simulink model "ML_UAV_3D_2"  (R2018a)
settings: Solver=ode4  StartTime=0.0  StopTime=130  FixedStep=Ts  MaxStep=2*T  MinStep=T  RelTol=1e-4
values from neighbouring files (symbols this model uses):
  Ac = 0.0331    [init_ML_UAV_3D_2.m]
  Am1_LPF = sysd.denominator{1}    [init_ML_UAV_3D_2.m]
  Am2_LPF = sysd.denominator{1}    [init_ML_UAV_3D_2.m]
  Am_coup_LPF = sysd.denominator{1}    [init_ML_UAV_3D_2.m]
  Amp_sf = 3    [init_ML_UAV_3D_2.m]
  Amp_sf_rp = 0.05*uav.m*g    [init_ML_UAV_3D_2.m]
  Bm1_LPF = sysd.numerator{1}    [init_ML_UAV_3D_2.m]
  Bm2_LPF = sysd.numerator{1}    [init_ML_UAV_3D_2.m]
  Bm_coup_LPF = sysd.numerator{1}    [init_ML_UAV_3D_2.m]
  C_S = [5;5;9]*10^-3    [init_ML_UAV_3D_2.m]
  Cd_u = 0.2    [init_ML_UAV_3D_2.m]
  dc_M_p = 6.7    [init_ML_UAV_3D_2.m]
  eps_V = 0.5    [init_ML_UAV_3D_2.m]
  g = 9.81    [init_ML_UAV_3D_2.m]
  gamma_d_p = (2*0.3/0.03*2*0.2*12/4)/10    (= 2.4)    [init_ML_UAV_3D_2.m]
  k3 = 24    [init_ML_UAV_3D_2.m]
  k4 = 0.8    [init_ML_UAV_3D_2.m]
  min_sf = 5    [init_ML_UAV_3D_2.m]
  min_sf_rp = 0.35*uav.m*g    [init_ML_UAV_3D_2.m]
  OMEGA_FILTER_OUTER = 40    [estimation.m]
  T_init = 10    [init_ML_UAV_3D_2.m]
  Tc = 1/500    (= 0.002)    [estimation.m]
  Tg = 1/ 20    (= 0.05)    [estimation.m]
  Tn = 1/500    (= 0.002)    [estimation.m]
  Ts = 1/500    (= 0.002)    [estimation.m]    (also in init_ML_UAV_3D_2.m)
  Tsc = 1/100    (= 0.01)    [estimation.m]
  Tz = 1/500    (= 0.002)    [estimation.m]
  X_GPS_offset = [0.01 0.005]    [estimation.m]
undefined symbols (not defined in the file or in its folder): Am_HPF, Am_LPF, Am_LPF2, an1, an1_v, an2, an3, Bm_HPF, Bm_LPF, Bm_LPF2, bn1, bn1_v, bn2, bn3, buoy, cable, controller, current, D_b, DiscIntNeverNeededParam, F, filters, J_u, K, kd_t, kp_t, L, Light, magnitude, MIL, Phi0, Psi0, R_b, T, Theta0, theta_q_ini, tolerences, torque_corr, uav, Vol_b, water, wave, X0_u
libraries: simulink x48, simulink_extras x10, UAV_Control x4, dspmtrx3 x2, aerolibwind2 x2
(part 5 of 6)

== system ML_UAV_3D_2/Quadrotor+buoy/6-DOF equations of motion Earth frame/M_1-5/buoy inertia ==
  Rb : Inport
  Rb_T : Inport  Port=2
  Demux : Demux  Outputs=3
  Demux1 : Demux  Outputs=2
  M_ii{,1..3} (4 alike) : Scope
  Product1 : Product  Inputs=3  Multiplication=Matrix(*)
  Selector : Selector  NumberOfDimensions=2  InputPortWidth=3  IndexOptions=Index vector (dialog),Index vector (dialog)  Indices=[1],[1 2 3]  OutputSizes=1,1
  Selector1 : Selector  NumberOfDimensions=2  InputPortWidth=3  IndexOptions=Index vector (dialog),Index vector (dialog)  Indices=[2],[2 3]  OutputSizes=1,1
  Selector2 : Selector  NumberOfDimensions=2  InputPortWidth=3  IndexOptions=Index vector (dialog),Index vector (dialog)  Indices=[3],[3]  OutputSizes=1,1
  Sum : Sum  Inputs=|++
  added mass : Constant  Value=diag([a_ii(1), a_ii(2), a_ii(3)])
  rigid body mass : Constant  Value=diag([m_b,m_b,m_b])
  M11_I : Outport
  M22_I : Outport  Port=2
  M12_I : Outport  Port=3
  M13_I : Outport  Port=4
  M33_I : Outport  Port=5
  M23_I : Outport  Port=6
  wires:
  rigid body mass/1 -> Sum/1
  added mass/1 -> Sum/2
  Rb/1 -> Product1/1  "Rb"
  Sum/1 -> Product1/2  "Mb'"
  Selector2/1 -> M_ii2/1, M33_I/1
  Selector/1 -> M_ii/1, Demux/1
  Product1/1 -> Selector2/1, Selector1/1, M_ii3/1, Selector/1
  Selector1/1 -> M_ii1/1, Demux1/1
  Demux/1 -> M11_I/1
  Demux/2 -> M12_I/1
  Demux/3 -> M13_I/1
  Demux1/1 -> M22_I/1
  Demux1/2 -> M23_I/1
  Rb_T/1 -> Product1/3

== system ML_UAV_3D_2/Quadrotor+buoy/6-DOF equations of motion Earth frame/M_12/added mass ==
  theta : Inport
  Add1 : Sum
  Add2 : Sum
  Add3 : Sum  Inputs=+-
  Constant13 : Constant  Value=2
  Gain : Gain  Gain=2
  M11 : Constant  Value=m_b+a_ii(1)
  "M11 " : Constant  Value=m_b+a_ii(1)
  M11 1 : Constant  Value=m_b+a_ii(1)
  "M22 " : Constant  Value=m_b+a_ii(2)
  M22 1 : Constant  Value=m_b+a_ii(2)
  M_22 : Constant  Value=m_b+a_ii(2)
  Product{,6..8} (4 alike) : Product  Inputs=3
  Product9 : Product  Inputs=**/
  Trigonometric Function1 : Trigonometry  Operator=sincos
  Trigonometric Function2 : Trigonometry  Operator=sincos
  Trigonometric Function3 : Trigonometry
  M11_I : Outport
  M22_I : Outport  Port=2
  M12_I : Outport  Port=3
  wires:
  Gain/1 -> Trigonometric Function3/1
  "M11 "/1 -> Product7/1
  Constant13/1 -> Product9/3
  Product7/1 -> Add2/1
  Add3/1 -> Product9/2
  M11 1/1 -> Add3/2
  M11/1 -> Product6/3
  M22 1/1 -> Add3/1
  "M22 "/1 -> Product8/3
  Product/1 -> Add1/1
  Product6/1 -> Add1/2
  Add2/1 -> M22_I/1
  Product8/1 -> Add2/2
  Trigonometric Function1/2 -> Product6/2, Product6/1
  Trigonometric Function2/1 -> Product7/3, Product7/2
  Trigonometric Function2/2 -> Product8/1, Product8/2
  M_22/1 -> Product/1
  Trigonometric Function3/1 -> Product9/1
  Trigonometric Function1/1 -> Product/2, Product/3
  theta/1 -> Gain/1, Trigonometric Function2/1, Trigonometric Function1/1
  Product9/1 -> M12_I/1
  Add1/1 -> M11_I/1

== system ML_UAV_3D_2/Quadrotor+buoy/6-DOF equations of motion Earth frame/Quadrotor Dynamics Outer-Loop/Gu ==
  coupled : Inport
  Constant4 : Constant  Value=m_u
  Gain1 : Gain  Gain=g
  Ground : Ground
  Product : Product
  Vector Concatenate : Concatenate  NumInputs=3
  G : Outport
  wires:
  Product/1 -> Gain1/1
  Constant4/1 -> Product/2  "u2"
  coupled/1 -> Product/1
  Vector Concatenate/1 -> G/1
  Gain1/1 -> Vector Concatenate/3  "u2"
  Ground/1 -> Vector Concatenate/2, Vector Concatenate/1

== system ML_UAV_3D_2/Quadrotor+buoy/6-DOF equations of motion Earth frame/Quadrotor Dynamics Outer-Loop/Integrator while decoupled ==
  acc : Inport
  X dot init : Inport  Port=2
  X init : Inport  Port=3
  X123 : Inport  Port=4
  reset : Inport  Port=5
  Enable : EnablePort
  Bias : Bias  Bias=L
  Bias3 : Bias  Bias=-L
  Saturation Dynamic : simulink/Discontinuities/Saturation Dynamic  OutMin=[]  OutMax=[]  OutDataTypeStr=Inherit: Same as second input  OutDataType=fixdt(1, 16)  OutScaling=2^-10  DoSatur=off
  Selector : Selector  InputPortWidth=5  IndexOptions=Index vector (dialog)  Indices=[1 2 3]  OutputSizes=1
  Selector1 : Selector  InputPortWidth=5  IndexOptions=Index vector (dialog)  Indices=[1 2 3]  OutputSizes=1
  Vector Concatenate2 : Concatenate
  Xu : DiscreteIntegrator  IntegratorMethod=Integration: Backward Euler  ExternalReset=level  InitialConditionSource=external  InitialCondition=theta_q_ini  SampleTime=-1  LimitOutput=on  StateName=theta  ICPrevOutput=DiscIntNeverNeededParam  ICPrevScaledInput=DiscIntNeverNeededParam
  dot(Xu) : DiscreteIntegrator  IntegratorMethod=Integration: Backward Euler  gainval=1  ExternalReset=level  InitialConditionSource=external  SampleTime=-1  ICPrevOutput=DiscIntNeverNeededParam  ICPrevScaledInput=DiscIntNeverNeededParam
  theta u{1..10} (10 alike) : Scope
  "dot(Xu) " : Outport
  "Xu " : Outport  Port=2
  wires:
  X dot init/1 -> theta u5/1, dot(Xu)/3
  Xu/1 -> theta u6/1, Vector Concatenate2/1, Saturation Dynamic/2
  X init/1 -> theta u7/1, Xu/3
  Saturation Dynamic/1 -> Vector Concatenate2/2, "Xu "/1
  X123/1 -> Selector/1, Selector1/1
  Selector/1 -> Bias/1
  Bias3/1 -> theta u10/1, Saturation Dynamic/3
  Vector Concatenate2/1 -> theta u3/1
  Bias/1 -> Saturation Dynamic/1, theta u9/1
  dot(Xu)/1 -> Xu/1, theta u1/1, "dot(Xu) "/1
  reset/1 -> theta u2/1, dot(Xu)/2, Xu/2
  acc/1 -> theta u4/1, dot(Xu)/1
  Selector1/1 -> theta u8/1, Bias3/1

== system ML_UAV_3D_2/Quadrotor+buoy/6-DOF equations of motion Earth frame/Quadrotor Dynamics Outer-Loop/Subsystem ==
  u1 : Inport
  R_u_3 : Inport  Port=2
  Product1 : Product  Inputs=**  SaturateOnIntegerOverflow=on  InputSameDT=on  OutDataTypeStr=Inherit: Same as first input
  tau_u : Outport
  wires:
  Product1/1 -> tau_u/1
  R_u_3/1 -> Product1/1
  u1/1 -> Product1/2

== system ML_UAV_3D_2/Quadrotor+buoy/6-DOF equations of motion Earth frame/Quadrotor Dynamics Outer-Loop/get initial UAV states for the decoupled dynamics ==
  X : Inport
  Xdot : Inport  Port=2
  Trigger : TriggerPort  TriggerType=falling  VariantControl=Variant
  Xu_init : Outport
  Vu_init : Outport  Port=2
  wires:
  X/1 -> Xu_init/1
  Xdot/1 -> Vu_init/1

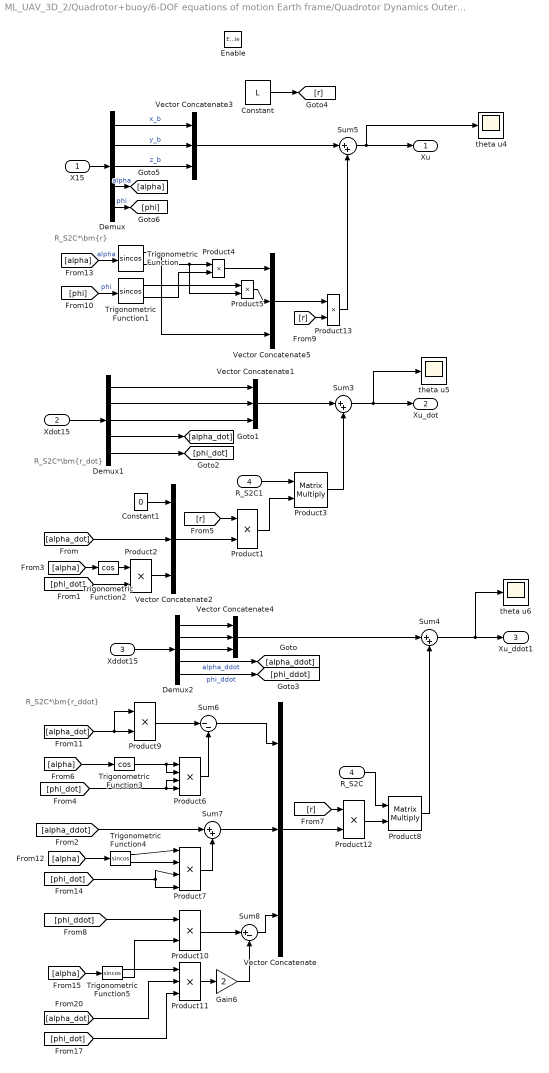
== system ML_UAV_3D_2/Quadrotor+buoy/6-DOF equations of motion Earth frame/Quadrotor Dynamics Outer-Loop/quadrotor position from relative buoy-UAV position ==
  note: R_S2C*\bm{r_ddot}
  note: R_S2C*\bm{r_dot}
  note: R_S2C*\bm{r}
  X15 : Inport
  Xdot15 : Inport  Port=2
  Xddot15 : Inport  Port=3
  R_S2C : Inport  Port=4
  Enable : EnablePort
  Constant : Constant  Value=L
  Constant1 : Constant  Value=0
  Demux : Demux  Outputs=5
  Demux1 : Demux  Outputs=5
  Demux2 : Demux  Outputs=5
  Gain6 : Gain  Gain=2
  Product{1..2,4..5,9..10,12..13} (8 alike) : Product
  Product11 : Product  Inputs=3
  Product3 : Product  Multiplication=Matrix(*)
  Product6 : Product  Inputs=4
  Product7 : Product  Inputs=4
  Product8 : Product  Multiplication=Matrix(*)
  R_S2C1 : InportShadow  Port=4
  Sum{3..5,7} (4 alike) : Sum  Inputs=|++
  Sum6 : Sum  Inputs=|--
  Sum8 : Sum  Inputs=|+-
  Trigonometric Function{,1,4..5} (4 alike) : Trigonometry  Operator=sincos
  Trigonometric Function2 : Trigonometry  Operator=cos
  Trigonometric Function3 : Trigonometry  Operator=cos
  Vector Concatenate{,1..5} (6 alike) : Concatenate  NumInputs=3
  theta u4 : Scope
  theta u5 : Scope
  theta u6 : Scope
  Xu : Outport
  Xu_dot : Outport  Port=2
  Xu_ddot1 : Outport  Port=3
  wires:
  [alpha] -> Trigonometric Function/1  "alpha"
  Sum5/1 -> Xu/1, theta u4/1
  Trigonometric Function/2 -> Product5/2, Product4/1
  Demux/2 -> Vector Concatenate3/2  "y_b"
  X15/1 -> Demux/1
  Demux/1 -> Vector Concatenate3/1  "x_b"
  R_S2C1/1 -> Product3/1
  Xdot15/1 -> Demux1/1
  Demux1/1 -> Vector Concatenate1/1
  Sum3/1 -> Xu_dot/1, theta u5/1
  Demux1/3 -> Vector Concatenate1/3
  Xddot15/1 -> Demux2/1
  Demux2/4 -> [alpha_ddot]  "alpha_ddot"
  [alpha_dot] -> Vector Concatenate2/2
  Product1/1 -> Product3/2
  Sum4/1 -> theta u6/1, Xu_ddot1/1
  Demux2/1 -> Vector Concatenate4/1
  Demux2/2 -> Vector Concatenate4/2
  [phi] -> Trigonometric Function1/1  "phi"
  Trigonometric Function1/2 -> Product4/2
  Trigonometric Function1/1 -> Product5/1
  Demux2/3 -> Vector Concatenate4/3
  [phi_dot] -> Product11/3
  Sum7/1 -> Vector Concatenate/2
  Product10/1 -> Sum8/1
  Vector Concatenate/1 -> Product12/2
  [alpha_dot] -> Product11/2
  [alpha] -> Trigonometric Function4/1
  Product7/1 -> Sum7/2
  Sum6/1 -> Vector Concatenate/1
  Sum8/1 -> Vector Concatenate/3
  Product6/1 -> Sum6/2
  Product11/1 -> Gain6/1
  Trigonometric Function5/1 -> Product11/1
  [alpha] -> Trigonometric Function5/1
  Product9/1 -> Sum6/1
  [alpha] -> Trigonometric Function3/1
  Demux2/5 -> [phi_ddot]  "phi_ddot"
  Demux1/5 -> [phi_dot]
  Demux1/4 -> [alpha_dot]
  Demux1/2 -> Vector Concatenate1/2
  Constant/1 -> [r]
  [alpha_ddot] -> Sum7/1
  [phi_ddot] -> Product10/1
  Trigonometric Function5/2 -> Product10/2
  Gain6/1 -> Sum8/2
  [r] -> Product12/1
  [alpha_dot] -> Product9/2, Product9/1
  Trigonometric Function3/1 -> Product6/2, Product6/1
  [phi_dot] -> Product6/3, Product6/4
  Trigonometric Function4/1 -> Product7/1
  Trigonometric Function4/2 -> Product7/2
  [phi_dot] -> Product7/4, Product7/3
  Product12/1 -> Product8/2
  R_S2C/1 -> Product8/1
  Vector Concatenate4/1 -> Sum4/1
  Product8/1 -> Sum4/2
  Constant1/1 -> Vector Concatenate2/1
  Product2/1 -> Vector Concatenate2/3
  [phi_dot] -> Product2/2
  [alpha] -> Trigonometric Function2/1
  Trigonometric Function2/1 -> Product2/1
  [r] -> Product1/1
  Vector Concatenate2/1 -> Product1/2
  Vector Concatenate1/1 -> Sum3/1
  Product3/1 -> Sum3/2
  Demux/3 -> Vector Concatenate3/3  "z_b"
  Vector Concatenate3/1 -> Sum5/1
  Product13/1 -> Sum5/2
  Product4/1 -> Vector Concatenate5/1
  Product5/1 -> Vector Concatenate5/2
  Trigonometric Function/1 -> Vector Concatenate5/3
  Vector Concatenate5/1 -> Product13/1
  [r] -> Product13/2
  Demux/4 -> [alpha]  "alpha"
  Demux/5 -> [phi]  "phi"

== system ML_UAV_3D_2/Quadrotor+buoy/6-DOF equations of motion Earth frame/Rigid Body Torque Equations /Rotation Angles to Angular transformation matrix body to earth Rotation Order: ZXY ==
  R1,R2,R3 : Inport  PortDimensions=3
  Fcn1 : Fcn  Expr=0
  Fcn11 : Fcn  Expr=u(5)
  Fcn13 : Fcn  Expr=u(2)
  Fcn21 : Fcn  Expr=u(2)*u(1)/u(4)
  Fcn22 : Fcn  Expr=1
  Fcn23 : Fcn  Expr=-u(5)*u(1)/u(4)
  Fcn3 : Fcn  Expr=u(5)/u(4)
  Fcn32 : Fcn  Expr=0
  Fcn33 : Fcn  Expr=-u(2)/u(4)
  Mux : Mux  Inputs=2
  Subsystem : Subsystem
  sincos : Trigonometry  Operator=sincos
  T : Outport  PortDimensions=[3,3]
  wires:
  R1,R2,R3/1 -> sincos/1
  Subsystem/1(Out1) -> T/1
  sincos/1 -> Mux/1
  sincos/2 -> Mux/2
  Mux/1 -> Fcn22/1, Fcn33/1, Fcn21/1, Fcn11/1, Fcn32/1, Fcn13/1, Fcn23/1, Fcn3/1, Fcn1/1
  Fcn11/1 -> Subsystem/1(In1)
  Fcn21/1 -> Subsystem/2(In2)
  Fcn33/1 -> Subsystem/3(In3)
  Fcn32/1 -> Subsystem/4(In4)
  Fcn13/1 -> Subsystem/7(In7)
  Fcn22/1 -> Subsystem/5(In5)
  Fcn1/1 -> Subsystem/6(In6)
  Fcn23/1 -> Subsystem/8(In8)
  Fcn3/1 -> Subsystem/9(In9)

== system ML_UAV_3D_2/Quadrotor+buoy/6-DOF equations of motion Earth frame/Tension from UAV, X and r directions/Tension from UAV, z direction ==
  alpha : Inport
  euler_u : Inport  Port=2
  u1 : Inport  Port=3
  Xu_ddot : Inport  Port=4
  Enable : EnablePort  StatesWhenEnabling=reset
  Add3 : Sum  Inputs=+--
  Constant : Constant  Value=m_u*g
  Demux : Demux  Outputs=2
  Gain14 : Gain
  Gain15 : Gain  Gain=m_u
  Product12 : Product  Inputs=3
  Product9 : Product  Inputs=*/
  Trigonometric Function6 : Trigonometry
  Trigonometric Function8 : Trigonometry  Operator=cos
  "phi, theta" : Selector  InputPortWidth=3  IndexOptions=Index vector (dialog)  Indices=[1 2]  OutputSizes=1
  z_ddot : Selector  InputPortWidth=3  IndexOptions=Index vector (dialog)  Indices=3  OutputSizes=1
  "T, from z simple" : Outport
  wires:
  Product9/1 -> "T, from z simple"/1
  Add3/1 -> Product9/1
  Gain14/1 -> Add3/1
  Demux/1 -> Product12/1
  u1/1 -> Product12/3
  alpha/1 -> Trigonometric Function6/1
  Product12/1 -> Gain14/1
  z_ddot/1 -> Gain15/1
  Trigonometric Function6/1 -> Product9/2
  Xu_ddot/1 -> z_ddot/1
  euler_u/1 -> "phi, theta"/1
  Gain15/1 -> Add3/2
  Constant/1 -> Add3/3
  Trigonometric Function8/1 -> Demux/1
  "phi, theta"/1 -> Trigonometric Function8/1
  Demux/2 -> Product12/2

== system ML_UAV_3D_2/Quadrotor+buoy/6-DOF equations of motion Earth frame/azimuthal dynamics/Coupled System's azimuthal dynamics ==
  "alpha, phi dc" : Inport
  "alpha_dot, phi _dot dc" : Inport  Port=2
  coupled : Inport  Port=3
  alpha_phi_ddot : Inport  Port=4
  recouple : Inport  Port=5
    alpha{,1..5} (6 alike) : Scope
  Clock : Clock
  Constant : Constant  Value=0
  Delay : Delay  DelayLength=1
  IC1 : InitialCondition  Value=a_p_0
  IC2 : InitialCondition  Value=0
  IC3 : InitialCondition  Value=a_p_0
  Logical Operator1 : Logic  Operator=NOT  AllPortsSameDT=off  OutDataTypeStr=boolean
  Switch : Switch  Criteria=u2 > Threshold  Threshold=2*Ts
  "T, r,xu,xb1" : Scope
  "T, r,xu,xb9" : Scope
  elevation and azimuth angles dynamics in the coupled system : Subsystem  TreatAsAtomicUnit=on
  get initial elevation and azimuth angle for the coupled dynamics : Subsystem  TreatAsAtomicUnit=on
  "alpha, phi coupled" : Outport
  "alpha_dot, phi_dot coupled" : Outport  Port=2
  wires:
  alpha_phi_ddot/1 -> elevation and azimuth angles dynamics in the coupled system/1(alpha_phi_ddot)
  coupled/1 -> elevation and azimuth angles dynamics in the coupled system/Enable, Logical Operator1/1
  elevation and azimuth angles dynamics in the coupled system/1("alpha, phi ") -> IC3/1
  elevation and azimuth angles dynamics in the coupled system/2("alpha_dot, phi_dot") -> "alpha_dot, phi_dot coupled"/1
  "alpha, phi dc"/1 -> "  alpha2"/1, get initial elevation and azimuth angle for the coupled dynamics/1("alpha, phi decoupled")
  "alpha_dot, phi _dot dc"/1 -> "  alpha1"/1, get initial elevation and azimuth angle for the coupled dynamics/2("alpha_dot, phi_dot decoupled")
  get initial elevation and azimuth angle for the coupled dynamics/1("alpha, phi init") -> "  alpha3"/1, IC1/1
  IC1/1 -> "  alpha4"/1, elevation and azimuth angles dynamics in the coupled system/2(alpha phi init)
  IC2/1 -> "  alpha5"/1, elevation and azimuth angles dynamics in the coupled system/3(alpha_phi_dot init)
  get initial elevation and azimuth angle for the coupled dynamics/2("alpha_dot, phi_dot init") -> IC2/1
  recouple/1 -> "  alpha"/1, get initial elevation and azimuth angle for the coupled dynamics/Trigger
  Logical Operator1/1 -> Delay/1
  Delay/1 -> Switch/1, "T, r,xu,xb1"/1
  Clock/1 -> Switch/2
  Switch/1 -> "T, r,xu,xb9"/1, elevation and azimuth angles dynamics in the coupled system/4(reset)
  Constant/1 -> Switch/3
  IC3/1 -> "alpha, phi coupled"/1

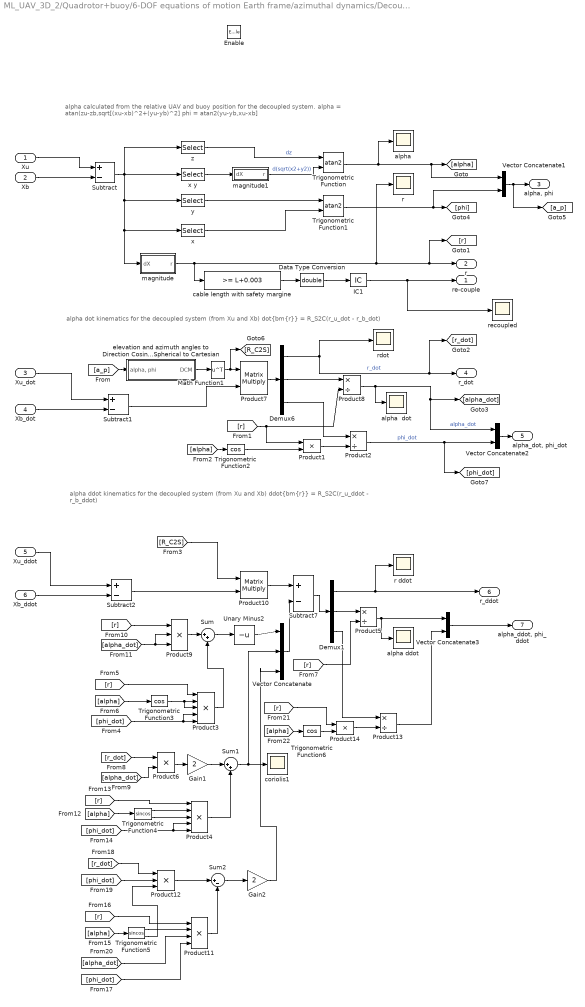
== system ML_UAV_3D_2/Quadrotor+buoy/6-DOF equations of motion Earth frame/azimuthal dynamics/Decoupled System's elevation and azimuth dynamics ==
  note: alpha dot kinematics for the decoupled system (from Xu and Xb)
      | dot{bm{r}} =  R_S2C(r_u_dot - r_b_dot)
  note: alpha calculated from the relative UAV and buoy position for the decoupled system.
      | alpha = atan(zu-zb,sqrt[(xu-xb)^2+(yu-yb)^2]
      | phi     = atan2(yu-yb,xu-xb]
  note: alpha ddot kinematics for the decoupled system (from Xu and Xb)
      | ddot{bm{r}} =  R_S2C(r_u_ddot - r_b_ddot)
  Xu : Inport
  Xb : Inport  Port=2
  Xu_dot : Inport  Port=3
  Xb_dot : Inport  Port=4
  Xu_ddot : Inport  Port=5
  Xb_ddot : Inport  Port=6
  Enable : EnablePort
  " r" : Scope
  Data Type Conversion : DataTypeConversion  OutDataTypeStr=double
  Demux1 : Demux  Outputs=3
  Demux6 : Demux  Outputs=3
  Gain1 : Gain  Gain=2
  Gain2 : Gain  Gain=2
  IC1 : InitialCondition  Value=0
  Math Function1 : Math  Operator=transpose  SaturateOnIntegerOverflow=on
  Product1 : Product
  Product10 : Product  Multiplication=Matrix(*)
  Product11 : Product  Inputs=4
  Product12 : Product  Inputs=3
  Product{2,5,8,13} (4 alike) : Product  Inputs=*/
  Product14 : Product
  Product3 : Product  Inputs=5
  Product4 : Product  Inputs=5
  Product6 : Product
  Product7 : Product  Multiplication=Matrix(*)
  Product9 : Product  Inputs=3
  Subtract{,1..2,7} (4 alike) : Sum  Inputs=+-
  Sum : Sum  Inputs=|++
  Sum1 : Sum  Inputs=|++
  Sum2 : Sum  Inputs=|+-
  Trigonometric Function : Trigonometry  Operator=atan2
  Trigonometric Function1 : Trigonometry  Operator=atan2
  Trigonometric Function2 : Trigonometry  Operator=cos
  Trigonometric Function3 : Trigonometry  Operator=cos
  Trigonometric Function4 : Trigonometry  Operator=sincos
  Trigonometric Function5 : Trigonometry  Operator=sincos
  Trigonometric Function6 : Trigonometry  Operator=cos
  Unary Minus2 : UnaryMinus
  Vector Concatenate : Concatenate  NumInputs=3
  Vector Concatenate1 : Concatenate
  Vector Concatenate2 : Concatenate
  Vector Concatenate3 : Concatenate
  "alpha     " : Scope
  alpha  dot : Scope
  alpha ddot : Scope
  cable length with safety margine : simulink/Logic and Bit Operations/Compare To Constant  relop=>=  const=L+0.003  OutDataTypeStr=boolean
  coriolis1 : Scope
  elevation and azimuth angles to Direction Cosine Matrix Spherical to Cartesian : Subsystem
      mask Display:
      | port_label('input',1,'\alpha, \phi','texmode','on')
      | port_label('output',1,'DCM_{S2C}','texmode','on')
  magnitude : Subsystem
  magnitude1 : Subsystem
  r ddot : Scope
  rdot : Scope
  recoupled : Scope
  x : Selector  InputPortWidth=3  IndexOptions=Index vector (dialog)  Indices=1  OutputSizes=1
  x y : Selector  InputPortWidth=3  IndexOptions=Index vector (dialog)  Indices=[1 2]  OutputSizes=1
  y : Selector  InputPortWidth=3  IndexOptions=Index vector (dialog)  Indices=2  OutputSizes=1
  z : Selector  InputPortWidth=3  IndexOptions=Index vector (dialog)  Indices=3  OutputSizes=1
  re-couple : Outport  OutputWhenDisabled=reset  InitialOutput=0
  r : Outport  Port=2
  "alpha, phi" : Outport  Port=3
  r_dot : Outport  Port=4
  "alpha_dot, phi_dot" : Outport  Port=5
  r_ddot : Outport  Port=6
  "alpha_ddot, phi_ddot" : Outport  Port=7
  wires:
  Xu_dot/1 -> Subtract1/1
  Xb_dot/1 -> Subtract1/2
  Xu/1 -> Subtract/1
  Xb/1 -> Subtract/2
  z/1 -> Trigonometric Function/1  "dz"
  magnitude1/1(r) -> Trigonometric Function/2  "d(sqrt(x2+y2))"
  Trigonometric Function/1 -> [alpha], Vector Concatenate1/1, "alpha     "/1
  Xu_ddot/1 -> Subtract2/1
  magnitude/1(r) -> " r"/1, [r], r/1, cable length with safety margine/1
  Subtract/1 -> z/1, x/1, magnitude/1(dX), y/1, x y/1
  cable length with safety margine/1 -> Data Type Conversion/1
  Data Type Conversion/1 -> IC1/1
  IC1/1 -> recoupled/1, re-couple/1
  [a_p] -> elevation and azimuth angles to Direction Cosine Matrix Spherical to Cartesian/1("alpha, phi")
  elevation and azimuth angles to Direction Cosine Matrix Spherical to Cartesian/1(DCM) -> Math Function1/1
  Subtract1/1 -> Product7/2
  Math Function1/1 -> [R_C2S], Product7/1
  Product7/1 -> Demux6/1
  Demux6/2 -> Product8/1
  [r] -> Product1/1, Product8/2
  Product8/1 -> alpha  dot/1, Vector Concatenate2/1, [alpha_dot]  "alpha_dot"
  Demux6/1 -> [r_dot], r_dot/1, rdot/1  "r_dot"
  Sum1/1 -> coriolis1/1, Vector Concatenate/2
  [r_dot] -> Product6/1
  [alpha_dot] -> Product6/2
  Product6/1 -> Gain1/1
  [r] -> Product5/2
  Xb_ddot/1 -> Subtract2/2
  Subtract2/1 -> Product10/2
  [R_C2S] -> Product10/1
  [r] -> Product9/1
  [alpha_dot] -> Product9/2, Product9/3
  Sum/1 -> Unary Minus2/1
  Product10/1 -> Subtract7/1
  Unary Minus2/1 -> Vector Concatenate/1
  Vector Concatenate/1 -> Subtract7/2
  Subtract7/1 -> Demux1/1
  Demux1/1 -> r ddot/1, r_ddot/1
  Demux1/2 -> Product5/1
  Product5/1 -> Vector Concatenate3/1, alpha ddot/1
  x y/1 -> magnitude1/1(dX)
  y/1 -> Trigonometric Function1/1
  x/1 -> Trigonometric Function1/2
  Trigonometric Function1/1 -> Vector Concatenate1/2, [phi]
  Vector Concatenate1/1 -> [a_p], "alpha, phi"/1
  [alpha] -> Trigonometric Function2/1
  Trigonometric Function2/1 -> Product1/2
  Product1/1 -> Product2/2
  Demux6/3 -> Product2/1
  Vector Concatenate2/1 -> "alpha_dot, phi_dot"/1
  Product2/1 -> [phi_dot], Vector Concatenate2/2  "phi_dot"
  [alpha] -> Trigonometric Function3/1
  [r] -> Product3/1
  Trigonometric Function3/1 -> Product3/3, Product3/2
  [phi_dot] -> Product3/4, Product3/5
  Product9/1 -> Sum/1
  Product3/1 -> Sum/2
  Gain1/1 -> Sum1/1
  [alpha] -> Trigonometric Function4/1
  Trigonometric Function4/1 -> Product4/2
  Trigonometric Function4/2 -> Product4/3
  [r] -> Product4/1
  [phi_dot] -> Product4/4, Product4/5
  Product4/1 -> Sum1/2
  Product11/1 -> Sum2/2
  [r] -> Product11/1
  Trigonometric Function5/2 -> Product12/3
  Trigonometric Function5/1 -> Product11/2
  [alpha] -> Trigonometric Function5/1
  Product12/1 -> Sum2/1
  [phi_dot] -> Product12/2
  [r_dot] -> Product12/1
  Sum2/1 -> Gain2/1
  [alpha_dot] -> Product11/3
  [phi_dot] -> Product11/4
  Gain2/1 -> Vector Concatenate/3
  Demux1/3 -> Product13/1
  [r] -> Product14/1
  Trigonometric Function6/1 -> Product14/2
  Product14/1 -> Product13/2
  [alpha] -> Trigonometric Function6/1
  Vector Concatenate3/1 -> "alpha_ddot, phi_ddot"/1
  Product13/1 -> Vector Concatenate3/2

== system ML_UAV_3D_2/Quadrotor+buoy/6-DOF equations of motion Earth frame/buoyancy/V_im cuboid ==
  zeta : Inport
  zb : Inport  Port=2
  Constant : Constant  Value=l_b*h_b
  Product3 : Product  SaturateOnIntegerOverflow=on  InputSameDT=on  OutDataTypeStr=Inherit: Same as first input
  Saturation : Saturate  UpperLimit=h_b/2  LowerLimit=-h_b/2
  Scope4 : Scope
  Sum : Sum  Inputs=|++
  Sum2 : Sum  Inputs=|+-  SaturateOnIntegerOverflow=on
  Vol_b/2 : Constant  Value=l_b*h_b*h_b/2
  Vol_im : Outport
  wires:
  Saturation/1 -> Product3/1
  Sum2/1 -> Saturation/1, Scope4/1  "d"
  Product3/1 -> Sum/1
  Constant/1 -> Product3/2
  Sum/1 -> Vol_im/1
  Vol_b/2/1 -> Sum/2
  zeta/1 -> Sum2/1
  zb/1 -> Sum2/2

== system ML_UAV_3D_2/Quadrotor+buoy/6-DOF equations of motion Earth frame/buoyancy/f(z_b,zeta) cylinder ==
  note: This model is valid for d<=R
  zeta : Inport
  zb : Inport  Port=2
  Bias : Bias  Bias=1
  Constant : Constant  Value=R_b
  Product3 : Product  Inputs=*/  SaturateOnIntegerOverflow=on  InputSameDT=on  OutDataTypeStr=Inherit: Same as first input
  Product4 : Product  SaturateOnIntegerOverflow=on  InputSameDT=on  OutDataTypeStr=Inherit: Same as first input
  Product5 : Product  SaturateOnIntegerOverflow=on  InputSameDT=on  OutDataTypeStr=Inherit: Same as first input
  Product6 : Product  SaturateOnIntegerOverflow=on  InputSameDT=on  OutDataTypeStr=Inherit: Same as first input
  Saturation : Saturate  UpperLimit=R_b  LowerLimit=0
  Scope{1..4} (4 alike) : Scope
  Sqrt : Sqrt  SaturateOnIntegerOverflow=on
  Sum2 : Sum  Inputs=-+|  SaturateOnIntegerOverflow=on
  Sum3 : Sum  Inputs=-+|  SaturateOnIntegerOverflow=on
  Unary Minus : UnaryMinus
  acos : Trigonometry  Operator=acos
  Out1 : Outport
  wires:
  Constant/1 -> Product5/2, Product3/2
  Bias/1 -> Sqrt/1
  Product5/1 -> Scope1/1, Sum3/2
  Product4/1 -> Sum3/1
  Product6/1 -> Unary Minus/1
  Unary Minus/1 -> Bias/1
  Sum2/1 -> Scope4/1, Saturation/1  "d"
  Product3/1 -> acos/1, Product6/2, Product6/1
  Sqrt/1 -> Product4/1, Scope3/1
  acos/1 -> Product5/1
  zb/1 -> Sum2/2
  zeta/1 -> Sum2/1
  Sum3/1 -> Out1/1
  Saturation/1 -> Scope2/1, Product4/2, Product3/1

== system ML_UAV_3D_2/Quadrotor+buoy/6-DOF equations of motion Earth frame/elevation and azimuth angles to Direction Cosine Matrix Spherical to Cartesian/Subsystem ==
  In1 : Inport
  In2 : Inport  Port=2
  In3 : Inport  Port=3
  In4 : Inport  Port=4
  In5 : Inport  Port=5
  In6 : Inport  Port=6
  In7 : Inport  Port=7
  In8 : Inport  Port=8
  In9 : Inport  Port=9
  Matrix Concatenate : Concatenate  NumInputs=3  Mode=Multidimensional array  ConcatenateDimension=2
  Mux : Mux  Inputs=3
  Mux1 : Mux  Inputs=3
  Mux2 : Mux  Inputs=3
  Reshape : Reshape  OutputDimensionality=Column vector (2-D)
  Reshape1 : Reshape  OutputDimensionality=Column vector (2-D)
  Reshape2 : Reshape  OutputDimensionality=Column vector (2-D)
  Out1 : Outport
  wires:
  Reshape1/1 -> Matrix Concatenate/2
  Mux1/1 -> Reshape1/1
  Reshape/1 -> Matrix Concatenate/1
  Reshape2/1 -> Matrix Concatenate/3
  Matrix Concatenate/1 -> Out1/1
  Mux2/1 -> Reshape2/1
  In1/1 -> Mux/1
  Mux/1 -> Reshape/1
  In4/1 -> Mux/2
  In7/1 -> Mux/3
  In2/1 -> Mux1/1
  In8/1 -> Mux1/3
  In5/1 -> Mux1/2
  In3/1 -> Mux2/1
  In6/1 -> Mux2/2
  In9/1 -> Mux2/3

== system ML_UAV_3D_2/Sensors and Filters/Data processing/Estimate Attitude/Calculate Roll and Pitch (From Acceleration Data) ==
  accel (m/s^2) [3] : Inport
  Gain1 : Gain  Commented=on  Gain=180/pi
  Gain3 : Gain
  Terminator : Terminator
  calc_roll_pitch : MATLAB Function  TreatAsAtomicUnit=on
  pitch_acc : Scope  Commented=on
  pitch_acc (rad) : Outport
  wires:
  accel (m/s^2) [3]/1 -> calc_roll_pitch/1(acc_body)
  calc_roll_pitch/2(pitch_acc) -> Gain3/1, Gain1/1
  Gain1/1 -> pitch_acc/1
  Gain3/1 -> pitch_acc (rad)/1
  calc_roll_pitch/1(roll_acc) -> Terminator/1

== system ML_UAV_3D_2/Sensors and Filters/Data processing/Estimate Attitude/Notch Filter1 ==
  u : Inport
  LPF : DiscreteTransferFcn  Numerator=Bm_LPF  Denominator=Am_LPF
  Mux : Mux  Commented=on
  Mux1 : Mux  Commented=on  Inputs=2
  Notch filter 1 : DiscreteTransferFcn  Numerator=an1  Denominator=bn1  SampleTime=Tn
  Notch filter 2 : DiscreteTransferFcn  Numerator=an2  Denominator=bn2  SampleTime=Tn
  Notch filter 3 : DiscreteTransferFcn  Numerator=an3  Denominator=bn3  SampleTime=Tn
  Scope : Scope  Commented=on
  Scope1 : Scope  Commented=on
  To File : ToFile  Commented=on  Filename=P_gyro_Noisy.mat  MatrixName=P_gyro_Noisy  SaveFormat=Timeseries
  y : Outport
  q : Outport  Port=2
  wires:
  u/1 -> Mux1/1, To File/1, LPF/1
  Notch filter 2/1 -> Mux/3, Notch filter 3/1
  LPF/1 -> Mux1/2, y/1, Notch filter 1/1, Mux/1
  Mux/1 -> Scope/1
  Notch filter 3/1 -> Mux/4, q/1
  Notch filter 1/1 -> Mux/2, Notch filter 2/1
  Mux1/1 -> Scope1/1

== system ML_UAV_3D_2/Sensors and Filters/Data processing/Estimate Position/2nd Order Filter ==
  u : Inport
  "  2" : Constant  Value=2
  "  wn" : Constant  Value=OMEGA_FILTER_OUTER
  "  zea" : Constant
  Discrete-Time Integrator : DiscreteIntegrator  SampleTime=-1  ICPrevOutput=DiscIntNeverNeededParam  ICPrevScaledInput=DiscIntNeverNeededParam
  Discrete-Time Integrator1 : DiscreteIntegrator  InitialCondition=X0_u(1)  SampleTime=-1  ICPrevOutput=DiscIntNeverNeededParam  ICPrevScaledInput=DiscIntNeverNeededParam
  Product : Product
  Product1 : Product
  Product2 : Product  Inputs=3
  Sum : Sum  Inputs=|+-
  Sum1 : Sum  Inputs=|+-
  y : Outport
  yd : Outport  Port=2
  wires:
  Sum/1 -> Sum1/1
  Discrete-Time Integrator/1 -> Product2/1, Product1/2
  Product/1 -> Discrete-Time Integrator/1
  "  wn"/1 -> Product1/1, Product/1
  Sum1/1 -> Product/2
  u/1 -> Sum/1
  Discrete-Time Integrator1/1 -> Sum/2, y/1
  Product1/1 -> Discrete-Time Integrator1/1, yd/1
  "  2"/1 -> Product2/2
  "  zea"/1 -> Product2/3
  Product2/1 -> Sum1/2

== system ML_UAV_3D_2/Sensors and Filters/Data processing/Estimate Position/2nd Order Filter2 ==
  u : Inport
  "  2" : Constant  Value=2
  "  wn" : Constant  Value=OMEGA_FILTER_OUTER
  "  zea" : Constant
  Discrete-Time Integrator : DiscreteIntegrator  SampleTime=-1  ICPrevOutput=DiscIntNeverNeededParam  ICPrevScaledInput=DiscIntNeverNeededParam
  Discrete-Time Integrator1 : DiscreteIntegrator  InitialCondition=X0_u(2)  SampleTime=-1  ICPrevOutput=DiscIntNeverNeededParam  ICPrevScaledInput=DiscIntNeverNeededParam
  Product : Product
  Product1 : Product
  Product2 : Product  Inputs=3
  Sum : Sum  Inputs=|+-
  Sum1 : Sum  Inputs=|+-
  y : Outport
  yd : Outport  Port=2
  wires:
  Sum/1 -> Sum1/1
  Discrete-Time Integrator/1 -> Product2/1, Product1/2
  Product/1 -> Discrete-Time Integrator/1
  "  wn"/1 -> Product1/1, Product/1
  Sum1/1 -> Product/2
  u/1 -> Sum/1
  Discrete-Time Integrator1/1 -> Sum/2, y/1
  Product1/1 -> Discrete-Time Integrator1/1, yd/1
  "  2"/1 -> Product2/2
  "  zea"/1 -> Product2/3
  Product2/1 -> Sum1/2

== system ML_UAV_3D_2/Sensors and Filters/Data processing/Estimate Position/2nd Order Filter4 ==
  u : Inport
  "  1" : Constant  Value=OMEGA_FILTER_OUTER
  "  2" : Constant  Value=2
  "  zea" : Constant
  Discrete-Time Integrator : DiscreteIntegrator  SampleTime=-1  ICPrevOutput=DiscIntNeverNeededParam  ICPrevScaledInput=DiscIntNeverNeededParam
  Discrete-Time Integrator1 : DiscreteIntegrator  InitialCondition=X0_u(2)  SampleTime=-1  ICPrevOutput=DiscIntNeverNeededParam  ICPrevScaledInput=DiscIntNeverNeededParam
  Product : Product
  Product1 : Product
  Product2 : Product  Inputs=3
  Sum : Sum  Inputs=|+-
  Sum1 : Sum  Inputs=|+-
  y : Outport
  yd : Outport  Port=2
  wires:
  Product2/1 -> Sum1/2
  "  zea"/1 -> Product2/3
  "  2"/1 -> Product2/2
  Product1/1 -> Discrete-Time Integrator1/1, yd/1
  Discrete-Time Integrator1/1 -> y/1, Sum/2
  u/1 -> Sum/1
  Sum1/1 -> Product/2
  "  1"/1 -> Product/1, Product1/1
  Product/1 -> Discrete-Time Integrator/1
  Discrete-Time Integrator/1 -> Product1/2, Product2/1
  Sum/1 -> Sum1/1

== system ML_UAV_3D_2/Sensors and Filters/Data processing/Estimate Position/2nd Order Filter5 ==
  u : Inport
  "  2" : Constant  Value=2
  "  wn" : Constant  Value=OMEGA_FILTER_OUTER
  "  zea" : Constant
  Discrete-Time Integrator : DiscreteIntegrator  SampleTime=-1  ICPrevOutput=DiscIntNeverNeededParam  ICPrevScaledInput=DiscIntNeverNeededParam
  Discrete-Time Integrator1 : DiscreteIntegrator  InitialCondition=X0_u(2)  SampleTime=-1  ICPrevOutput=DiscIntNeverNeededParam  ICPrevScaledInput=DiscIntNeverNeededParam
  Product : Product
  Product1 : Product
  Product2 : Product  Inputs=3
  Sum : Sum  Inputs=|+-
  Sum1 : Sum  Inputs=|+-
  y : Outport
  yd : Outport  Port=2
  wires:
  Product2/1 -> Sum1/2
  "  zea"/1 -> Product2/3
  "  2"/1 -> Product2/2
  Product1/1 -> Discrete-Time Integrator1/1, yd/1
  Discrete-Time Integrator1/1 -> y/1, Sum/2
  u/1 -> Sum/1
  Sum1/1 -> Product/2
  "  wn"/1 -> Product/1, Product1/1
  Product/1 -> Discrete-Time Integrator/1
  Discrete-Time Integrator/1 -> Product1/2, Product2/1
  Sum/1 -> Sum1/1

== system ML_UAV_3D_2/Sensors and Filters/Data processing/Estimate Position/Notch Filter2 ==
  u : Inport
  LPF : DiscreteTransferFcn  Numerator=Bm_LPF  Denominator=Am_LPF
  Mux : Mux  Commented=on  Inputs=3
  Notch filter : DiscreteTransferFcn  Numerator=an1_v  Denominator=bn1_v  SampleTime=Tn
  Scope : Scope  Commented=on
  y : Outport
  wires:
  Notch filter/1 -> y/1, Mux/3
  Mux/1 -> Scope/1
  LPF/1 -> Mux/2, Notch filter/1
  u/1 -> LPF/1, Mux/1

== system ML_UAV_3D_2/Sensors and Filters/Data processing/Estimate Position/Signal Conditioning - Sonar ==
  note: Correct for Roll and Pitch
  sonar (m) : Inport
  pitch (rad) : Inport  Port=2
  "Height Estimate Bias (Estimate Reference at Centre of QBall 2) " : Bias
  Product : Product  RndMeth=Zero
  "The sonar signal is the true elevation, so no need for correction" : Constant
  Trigonometric Function : Trigonometry  Commented=on  Operator=cos
  calib sonar (m) : Outport
  wires:
  sonar (m)/1 -> Product/1
  pitch (rad)/1 -> Trigonometric Function/1
  "The sonar signal is the true elevation, so no need for correction"/1 -> Product/2
  Product/1 -> "Height Estimate Bias (Estimate Reference at Centre of QBall 2) "/1
  "Height Estimate Bias (Estimate Reference at Centre of QBall 2) "/1 -> calib sonar (m)/1

== system ML_UAV_3D_2/Sensors and Filters/Sensors/ Sonar (10Hz) (true elevation instead real sonar signal)/FOH1 ==
  Input : Inport
  Bias : Bias  Bias=-Ts
  Constant : Constant
  Digital Clock : DigitalClock  DisableCoverage=on  SampleTime=Ts
  Discrete-Time Integrator : DiscreteIntegrator  SampleTime=-1  ICPrevOutput=DiscIntNeverNeededParam  ICPrevScaledInput=DiscIntNeverNeededParam
  Gain : Gain  DisableCoverage=on  Gain=1/Ts  SaturateOnIntegerOverflow=on  OutDataTypeStr=Inherit: Same as input  ParamDataTypeStr=Inherit: Same as input
  Product : Product  RndMeth=Zero
  Rate Transition : RateTransition
  Rate Transition1 : RateTransition  OutPortSampleTime=T
  Rate Transition3 : RateTransition  OutPortSampleTime=T
  Rate Transition4 : RateTransition  InitialCondition=X0_u(2)  OutPortSampleTime=Ts
  Rate Transition5 : RateTransition  OutPortSampleTime=T
  Scope : Scope  Commented=on
  Scope1 : Scope  Commented=on
  Sum : Sum  DisableCoverage=on  Inputs=|+-  SaturateOnIntegerOverflow=on  InputSameDT=on  OutDataTypeStr=Inherit: Same as first input
  Sum2 : Sum  DisableCoverage=on  Inputs=|+-  SaturateOnIntegerOverflow=on  InputSameDT=on  OutDataTypeStr=Inherit: Same as first input
  Unit Delay : UnitDelay  DisableCoverage=on  InitialCondition=X0_u(2)  SampleTime=Ts
  s : Sum  Inputs=++|  SaturateOnIntegerOverflow=on  InputSameDT=on  OutDataTypeStr=Inherit: Same as first input
  Output : Outport
  wires:
  Input/1 -> Rate Transition4/1, Rate Transition5/1
  Unit Delay/1 -> Sum/2
  Rate Transition1/1 -> Scope1/1, Product/1
  Product/1 -> s/2
  Rate Transition3/1 -> Product/2, Scope/1
  Sum/1 -> Rate Transition1/1
  Bias/1 -> Sum2/1
  Discrete-Time Integrator/1 -> Bias/1
  Rate Transition/1 -> Sum2/2
  s/1 -> Output/1
  Rate Transition5/1 -> s/1
  Gain/1 -> Rate Transition3/1
  Digital Clock/1 -> Rate Transition/1
  Sum2/1 -> Gain/1
  Constant/1 -> Discrete-Time Integrator/1
  Rate Transition4/1 -> Sum/1, Unit Delay/1

== system ML_UAV_3D_2/Sensors and Filters/Sensors/ Sonar (10Hz) (true elevation instead real sonar signal)/Sampler ==
  In1 : Inport
  Constant : Constant  Value=X0_u(2)
  Derivative : Derivative
  Digital Clock : DigitalClock  DisableCoverage=on  SampleTime=0.1
  Rate Transition : RateTransition  InitialCondition=0.1
  Switch : Switch  Threshold=0.2
  Triggered Subsystem : Subsystem  TreatAsAtomicUnit=on
  Out1 : Outport
  wires:
  Derivative/1 -> Triggered Subsystem/Trigger
  Rate Transition/1 -> Derivative/1
  In1/1 -> Triggered Subsystem/1(In1)
  Switch/1 -> Out1/1
  Digital Clock/1 -> Switch/2, Rate Transition/1
  Triggered Subsystem/1(Out1) -> Switch/1
  Constant/1 -> Switch/3

== system ML_UAV_3D_2/UAV controller/u_r_p_Lyapunov radial position2/nu_x, buoy surge velocity controller/smooth switch ==
  note: if switch == 1
      | y = u1
      | elseif switch == 0
      | y = u2
      | end
  u 1 : Inport
  u 2 : Inport  Port=2
  switch : Inport  Port=3
  Constant : Constant
  Data Type Conversion : DataTypeConversion
  Low Pass Filter2 : DiscreteTransferFcn  Numerator=filters.Bm_coup_LPF  Denominator=filters.Am_coup_LPF
  Product : Product
  Product1 : Product
  Step1 : Step  SampleTime=0
  Subtract : Sum  Inputs=+-
  Sum : Sum  Inputs=|++
  "switch " : Scope
  y : Outport
  wires:
  Product/1 -> Sum/2
  Product1/1 -> Sum/1
  Low Pass Filter2/1 -> "switch "/1, Product/1, Subtract/2
  Data Type Conversion/1 -> Low Pass Filter2/1
  u 1/1 -> Product1/1
  u 2/1 -> Product/2
  switch/1 -> Data Type Conversion/1
  Sum/1 -> y/1
  Constant/1 -> Subtract/1
  Subtract/1 -> Product1/2

== system ML_UAV_3D_2/UAV controller/u_r_p_Lyapunov radial position2/output conditioning/Subsystem1 ==
  switch : Inport
  u_r : Inport  Port=2
  Switch4 : Switch  Criteria=u2 > Threshold
  "ur smooth lower bound, coupled" : Subsystem
  "ur smooth lower bound, decoupled" : Subsystem
  Out1 : Outport
  wires:
  "ur smooth lower bound, coupled"/1(sat(u)) -> Switch4/1
  u_r/1 -> "ur smooth lower bound, decoupled"/1(u), "ur smooth lower bound, coupled"/1(u)
  "ur smooth lower bound, decoupled"/1(sat(u)) -> Switch4/3
  Switch4/1 -> Out1/1
  switch/1 -> Switch4/2

== system ML_UAV_3D_2/UAV controller/u_r_p_Lyapunov radial position2/output conditioning/smooth lower bound2 ==
  u : Inport
  Manual Switch : ManualSwitch  CurrentSetting=0
  Mux3 : Mux  Inputs=2
  Saturation7 : Saturate  UpperLimit=5*g*uav.m  LowerLimit=-2*g*uav.m
  apply for lower bound only : Switch  Criteria=u2 > Threshold  Threshold=Amp_sf+min_sf
  sat : Scope
  saturation function : Fcn  Expr=Amp_sf*tanh((u(1)+(Amp_sf+min_sf))/(Amp_sf)) + (Amp_sf+min_sf)
  sat(u) : Outport
  wires:
  apply for lower bound only/1 -> Manual Switch/1
  Mux3/1 -> sat/1
  saturation function/1 -> Mux3/2, apply for lower bound only/3
  u/1 -> Saturation7/1, apply for lower bound only/1, Mux3/1, apply for lower bound only/2, saturation function/1
  Saturation7/1 -> Manual Switch/2
  Manual Switch/1 -> sat(u)/1

== system ML_UAV_3D_2/UAV controller/u_r_p_Lyapunov radial position2/output conditioning/smooth switching with memory ==
  note: The value of the signal at switching is held (not reset to zeo) so that the switching algorithm can work properly.
      | This block has a single vector input, and switches smoothly between the new values of the same vector at the desired time.
  u : Inport
  switch : Inport  Port=2
  Enabled Subsystem1 : Subsystem  TreatAsAtomicUnit=on
  Enabled Subsystem2 : Subsystem  TreatAsAtomicUnit=on
  Logical Operator : Logic  Operator=NOT  AllPortsSameDT=off  OutDataTypeStr=boolean
  smooth switch : Subsystem
  y : Outport
  wires:
  switch/1 -> smooth switch/3(switch), Logical Operator/1, Enabled Subsystem1/Enable
  Logical Operator/1 -> Enabled Subsystem2/Enable
  u/1 -> Enabled Subsystem1/1(In1), Enabled Subsystem2/1(In1)
  smooth switch/1(y) -> y/1
  Enabled Subsystem1/1(Out1) -> smooth switch/1(u 1)
  Enabled Subsystem2/1(Out1) -> smooth switch/2(u 2)

== system ML_UAV_3D_2/UAV controller/u_r_p_Lyapunov radial position2/u_alpha, both controllers/smooth switch ==
  note: if switch == 0
      | y = u2
      | elseif switch == 1
      | y = u1
      | end
  u 1 : Inport
  u 2 : Inport  Port=2
  switch : Inport  Port=3
  Constant : Constant
  Data Type Conversion : DataTypeConversion
  Low Pass Filter2 : DiscreteTransferFcn  Numerator=filters.Bm_coup_LPF  Denominator=filters.Am_coup_LPF
  Product : Product
  Product1 : Product
  Step1 : Step  SampleTime=0
  Subtract : Sum  Inputs=+-
  Sum : Sum  Inputs=|++
  "switch " : Scope
  y : Outport
  wires:
  Product/1 -> Sum/2
  Product1/1 -> Sum/1
  Low Pass Filter2/1 -> "switch "/1, Product/1, Subtract/2
  Data Type Conversion/1 -> Low Pass Filter2/1
  u 2/1 -> Product1/1
  u 1/1 -> Product/2
  switch/1 -> Data Type Conversion/1
  Sum/1 -> y/1
  Constant/1 -> Subtract/1
  Subtract/1 -> Product1/2

== system ML_UAV_3D_2/UAV controller/u_r_p_Lyapunov radial position2/u_alpha, both controllers1/smooth switch ==
  note: if switch == 0
      | y = u2
      | elseif switch == 1
      | y = u1
      | end
  u 1 : Inport
  u 2 : Inport  Port=2
  switch : Inport  Port=3
  Constant : Constant
  Data Type Conversion : DataTypeConversion
  Low Pass Filter2 : DiscreteTransferFcn  Numerator=filters.Bm_coup_LPF  Denominator=filters.Am_coup_LPF
  Product : Product
  Product1 : Product
  Step1 : Step  SampleTime=0
  Subtract : Sum  Inputs=+-
  Sum : Sum  Inputs=|++
  "switch " : Scope
  y : Outport
  wires:
  Product/1 -> Sum/2
  Product1/1 -> Sum/1
  Low Pass Filter2/1 -> "switch "/1, Product/1, Subtract/2
  Data Type Conversion/1 -> Low Pass Filter2/1
  u 2/1 -> Product1/1
  u 1/1 -> Product/2
  switch/1 -> Data Type Conversion/1
  Sum/1 -> y/1
  Constant/1 -> Subtract/1
  Subtract/1 -> Product1/2

== system ML_UAV_3D_2/UAV controller/u_r_p_Lyapunov radial position3/output conditioning/Subsystem1 ==
  switch : Inport
  u_r : Inport  Port=2
  Switch4 : Switch  Criteria=u2 > Threshold
  "ur smooth lower bound, coupled" : Subsystem
  "ur smooth lower bound, decoupled" : Subsystem
  Out1 : Outport
  wires:
  "ur smooth lower bound, coupled"/1(sat(u)) -> Switch4/1
  u_r/1 -> "ur smooth lower bound, decoupled"/1(u), "ur smooth lower bound, coupled"/1(u)
  "ur smooth lower bound, decoupled"/1(sat(u)) -> Switch4/3
  Switch4/1 -> Out1/1
  switch/1 -> Switch4/2

== system ML_UAV_3D_2/UAV controller/u_r_p_Lyapunov radial position3/output conditioning/smooth lower bound2 ==
  u : Inport
  Manual Switch : ManualSwitch  CurrentSetting=0
  Mux3 : Mux  Inputs=2
  Saturation7 : Saturate  UpperLimit=25*uav.m  LowerLimit=0
  apply for lower bound only : Switch  Criteria=u2 > Threshold  Threshold=Amp_sf+min_sf
  sat : Scope
  saturation function : Fcn  Expr=Amp_sf*tanh((u(1)+(Amp_sf+min_sf))/(Amp_sf)) + (Amp_sf+min_sf)
  sat(u) : Outport
  wires:
  apply for lower bound only/1 -> Manual Switch/1
  Mux3/1 -> sat/1
  saturation function/1 -> Mux3/2, apply for lower bound only/3
  u/1 -> Saturation7/1, apply for lower bound only/1, Mux3/1, apply for lower bound only/2, saturation function/1
  Saturation7/1 -> Manual Switch/2
  Manual Switch/1 -> sat(u)/1

== system ML_UAV_3D_2/UAV controller/u_r_p_Lyapunov radial position3/output conditioning/smooth switching with memory ==
  note: The value of the signal at switching is held (not reset to zeo) so that the switching algorithm can work properly.
      | This block has a single vector input, and switches smoothly between the new values of the same vector at the desired time.
  u : Inport
  switch : Inport  Port=2
  Enabled Subsystem1 : Subsystem  TreatAsAtomicUnit=on
  Enabled Subsystem2 : Subsystem  TreatAsAtomicUnit=on
  Logical Operator : Logic  Operator=NOT  AllPortsSameDT=off  OutDataTypeStr=boolean
  smooth switch : Subsystem
  y : Outport
  wires:
  switch/1 -> smooth switch/3(switch), Logical Operator/1, Enabled Subsystem1/Enable
  Logical Operator/1 -> Enabled Subsystem2/Enable
  u/1 -> Enabled Subsystem1/1(In1), Enabled Subsystem2/1(In1)
  smooth switch/1(y) -> y/1
  Enabled Subsystem1/1(Out1) -> smooth switch/1(u 1)
  Enabled Subsystem2/1(Out1) -> smooth switch/2(u 2)

== system ML_UAV_3D_2/UAV controller/u_r_p_Lyapunov radial position3/u_alpha, both controllers/smooth switch ==
  note: if switch == 0
      | y = u2
      | elseif switch == 1
      | y = u1
      | end
  u 1 : Inport
  u 2 : Inport  Port=2
  switch : Inport  Port=3
  Constant : Constant
  Data Type Conversion : DataTypeConversion
  Low Pass Filter2 : DiscreteTransferFcn  Numerator=Bm_coup_LPF  Denominator=Am_coup_LPF
  Product : Product
  Product1 : Product
  Step1 : Step  SampleTime=0
  Subtract : Sum  Inputs=+-
  Sum : Sum  Inputs=|++
  "switch " : Scope
  y : Outport
  wires:
  Product/1 -> Sum/2
  Product1/1 -> Sum/1
  Low Pass Filter2/1 -> "switch "/1, Product/1, Subtract/2
  Data Type Conversion/1 -> Low Pass Filter2/1
  u 2/1 -> Product1/1
  u 1/1 -> Product/2
  switch/1 -> Data Type Conversion/1
  Sum/1 -> y/1
  Constant/1 -> Subtract/1
  Subtract/1 -> Product1/2

== system ML_UAV_3D_2/UAV controller/u_r_p_Lyapunov radial position3/u_x, buoy surge velocity controller/smooth switch ==
  note: if switch == 1
      | y = u1
      | elseif switch == 0
      | y = u2
      | end
  u 1 : Inport
  u 2 : Inport  Port=2
  switch : Inport  Port=3
  Constant : Constant
  Data Type Conversion : DataTypeConversion
  Low Pass Filter2 : DiscreteTransferFcn  Numerator=Bm_coup_LPF  Denominator=Am_coup_LPF
  Product : Product
  Product1 : Product
  Step1 : Step  SampleTime=0
  Subtract : Sum  Inputs=+-
  Sum : Sum  Inputs=|++
  "switch " : Scope
  y : Outport
  wires:
  Product/1 -> Sum/2
  Product1/1 -> Sum/1
  Low Pass Filter2/1 -> "switch "/1, Product/1, Subtract/2
  Data Type Conversion/1 -> Low Pass Filter2/1
  u 1/1 -> Product1/1
  u 2/1 -> Product/2
  switch/1 -> Data Type Conversion/1
  Sum/1 -> y/1
  Constant/1 -> Subtract/1
  Subtract/1 -> Product1/2

== system ML_UAV_3D_2/UAV controller/u_r_p_Lyapunov radial position3/u_y, buoy surge velocity controller/smooth switch1 ==
  note: if switch == 1
      | y = u1
      | elseif switch == 0
      | y = u2
      | end
  u 1 : Inport
  u 2 : Inport  Port=2
  switch : Inport  Port=3
  Constant : Constant
  Data Type Conversion : DataTypeConversion
  Low Pass Filter2 : DiscreteTransferFcn  Numerator=Bm_coup_LPF  Denominator=Am_coup_LPF
  Product : Product
  Product1 : Product
  Subtract : Sum  Inputs=+-
  Sum : Sum  Inputs=|++
  "switch " : Scope
  y : Outport
  wires:
  Product/1 -> Sum/2
  Product1/1 -> Sum/1
  Low Pass Filter2/1 -> "switch "/1, Product/1, Subtract/2
  Data Type Conversion/1 -> Low Pass Filter2/1
  u 1/1 -> Product1/1
  u 2/1 -> Product/2
  switch/1 -> Data Type Conversion/1
  Sum/1 -> y/1
  Constant/1 -> Subtract/1
  Subtract/1 -> Product1/2

== system ML_UAV_3D_2/Quadrotor+buoy/6-DOF equations of motion Earth frame/D_1-5/Water Daming/buoy damping matric ==
  Rb : Inport
  Rb_T : Inport  Port=2
  D_b' : Inport  Port=3
  Constant : Constant  Commented=on  Value=diag([1 1 1])
  D_ii2 : Scope
  D_ii3 : Scope
  Demux1 : Demux  Outputs=3
  Demux2 : Demux  Outputs=2
  M : Scope
  M_ii 1 : Scope
  Product1 : Product  Inputs=3  Multiplication=Matrix(*)
  Selector : Selector  NumberOfDimensions=2  InputPortWidth=3  IndexOptions=Index vector (dialog),Index vector (dialog)  Indices=[1],[1 2 3]  OutputSizes=1,1
  Selector1 : Selector  NumberOfDimensions=2  InputPortWidth=3  IndexOptions=Index vector (dialog),Index vector (dialog)  Indices=[2],[2 3]  OutputSizes=1,1
  Selector2 : Selector  NumberOfDimensions=2  InputPortWidth=3  IndexOptions=Index vector (dialog),Index vector (dialog)  Indices=[3],[3]  OutputSizes=1,1
  D11_I : Outport
  D12_I : Outport  Port=2
  D13_I : Outport  Port=3
  D22_I : Outport  Port=4
  D23_I : Outport  Port=5
  D33_I : Outport  Port=6
  wires:
  Rb/1 -> Product1/1
  D_b'/1 -> Product1/2
  Selector1/1 -> D_ii2/1, Demux2/1
  Demux2/2 -> D23_I/1
  Demux2/1 -> D22_I/1
  Demux1/2 -> D12_I/1
  Product1/1 -> Selector2/1, Selector1/1, M/1, Selector/1
  Selector/1 -> M_ii 1/1, Demux1/1
  Selector2/1 -> D_ii3/1, D33_I/1
  Demux1/3 -> D13_I/1
  Demux1/1 -> D11_I/1
  Rb_T/1 -> Product1/3

== system ML_UAV_3D_2/Quadrotor+buoy/6-DOF equations of motion Earth frame/D_1-5/Water Daming (simplified/buoy damping ==
  euler_b : Inport
  D_b' : Inport  Port=2
  D_ii2 : Scope
  D_ii3 : Scope
  Demux : Demux  Outputs=9
  M : Scope
  M_ii 1 : Scope
  Math Function : Math  Operator=transpose  SaturateOnIntegerOverflow=on
  Product1 : Product  Inputs=3  Multiplication=Matrix(*)
  Rotation Angles to Direction Cosine Matrix body to earth Rotation Order: ZXY : UAV_Control/Rotation Angles to Direction Cosine Matrix body to earth Rotation Order: ZXY
      settings: SourceProductName=UAV_Control
  Terminator : Terminator
  Terminator1 : Terminator
  Terminator2 : Terminator
  D11_I : Outport
  D12_I : Outport  Port=2
  D13_I : Outport  Port=3
  D22_I : Outport  Port=4
  D23_I : Outport  Port=5
  D33_I : Outport  Port=6
  wires:
  Demux/1 -> M_ii 1/1, D11_I/1
  Demux/5 -> D_ii2/1, D22_I/1
  euler_b/1 -> Rotation Angles to Direction Cosine Matrix body to earth Rotation Order: ZXY/1
  Rotation Angles to Direction Cosine Matrix body to earth Rotation Order: ZXY/1 -> Math Function/1, Product1/1
  D_b'/1 -> Product1/2
  Math Function/1 -> Product1/3
  Demux/2 -> D12_I/1
  Demux/3 -> D13_I/1
  Demux/9 -> D_ii3/1, D33_I/1
  Demux/6 -> D23_I/1
  Demux/7 -> Terminator/1
  Demux/8 -> Terminator1/1
  Demux/4 -> Terminator2/1
  Product1/1 -> M/1, Demux/1

== system ML_UAV_3D_2/Quadrotor+buoy/6-DOF equations of motion Earth frame/Rigid Body Torque Equations /Rotation Angles to Angular transformation matrix body to earth Rotation Order: ZXY/Subsystem ==
  In1 : Inport
  In2 : Inport  Port=2
  In3 : Inport  Port=3
  In4 : Inport  Port=4
  In5 : Inport  Port=5
  In6 : Inport  Port=6
  In7 : Inport  Port=7
  In8 : Inport  Port=8
  In9 : Inport  Port=9
  Matrix Concatenate : Concatenate  NumInputs=3  Mode=Multidimensional array  ConcatenateDimension=2
  Mux : Mux  Inputs=3
  Mux1 : Mux  Inputs=3
  Mux2 : Mux  Inputs=3
  Reshape : Reshape  OutputDimensionality=Column vector (2-D)
  Reshape1 : Reshape  OutputDimensionality=Column vector (2-D)
  Reshape2 : Reshape  OutputDimensionality=Column vector (2-D)
  Out1 : Outport
  wires:
  In9/1 -> Mux2/3
  In8/1 -> Mux2/2
  In7/1 -> Mux2/1
  In6/1 -> Mux1/3
  In5/1 -> Mux1/2
  In4/1 -> Mux1/1
  In3/1 -> Mux/3
  In2/1 -> Mux/2
  In1/1 -> Mux/1
  Mux/1 -> Reshape/1
  Mux2/1 -> Reshape2/1
  Matrix Concatenate/1 -> Out1/1
  Reshape2/1 -> Matrix Concatenate/3
  Reshape/1 -> Matrix Concatenate/1
  Mux1/1 -> Reshape1/1
  Reshape1/1 -> Matrix Concatenate/2
